simulink model "washing_mac"  (R2024b)
settings: Solver=VariableStepAuto  StartTime=0.0  StopTime=inf  RelTol=1e-3
settings Model: Creator=Ajay1  LastModifiedBy=Ajay1

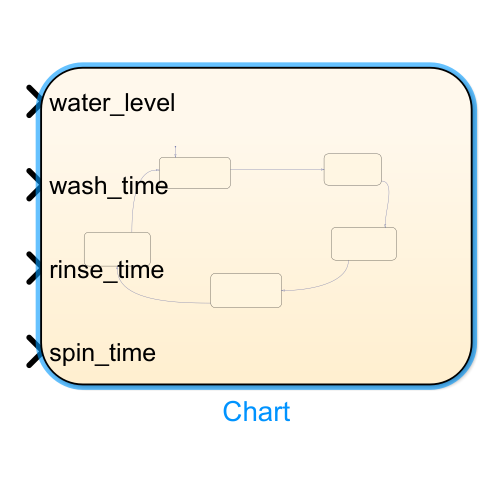
[thumbnail: Simulink's stored preview of the top-level diagram]
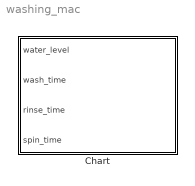
== system washing_mac ==
  Chart : Stateflow chart  TreatAsAtomicUnit=on

== stateflow chart washing_mac/Chart ==
  state run2
    entry:
    wash_timer=wash_timer+dt;
  state run1
    entry:
    water_level=water_level+fill_rate;
  state run3
    entry:
    rinse_time=rinse_time+dt;
  state done
  state run4
    entry:
    spin_time=spin_time+dt;
  (default) -> run1
  run1 -> run2 : [water_level>=threshold]
  done -> run1
  run2 -> run3 : [wash_time>=washduration]
  run3 -> run4 : [rinse_time>=rinse_duration]
  run4 -> done : [spin_time>=spin_duration]
  data: threshold constant double; spin_duration constant double; rinse_duration constant double; water_level input double; dt constant double; fill_rate constant double; washduration constant double; wash_timer constant double; wash_time input double; rinse_time input double; spin_time input double
